simulink model "2Zad_Adasiak"  (R2020b)
settings: Solver=VariableStepAuto  StartTime=0.0  StopTime=0.0  RelTol=1e-3
undefined symbols (not defined in the file): W
libraries: CPOiS_SourcesSinks x15, CPOiS_LinearTransforms x5, CPOiS_General x1
settings Model: Creator=Krystian  LastModifiedBy=Krystian

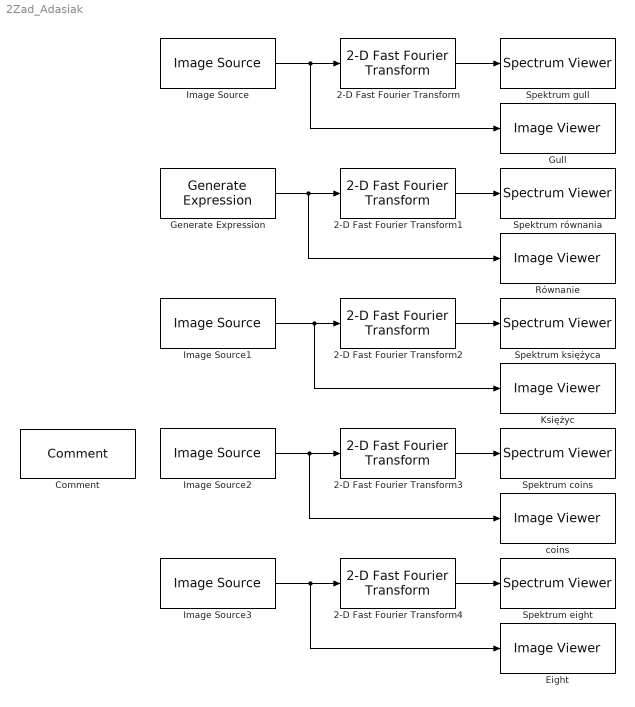
== system 2Zad_Adasiak ==
  2-D Fast Fourier Transform{,1..4} (5 alike) : CPOiS_LinearTransforms/2-D Fast Fourier Transform
      settings: SourceProductName=CPOiS - Digital image and signal processing
  Comment : CPOiS_General/Comment
      settings: SourceProductName=CPOiS - Digital image and signal processing
  Eight : CPOiS_SourcesSinks/Image Viewer
      settings: SourceProductName=CPOiS - Digital image and signal processing
  Generate Expression : CPOiS_SourcesSinks/Generate Expression  Width=256  Height=256  Expression=128.*(sin(W)+1)
      settings: SourceProductName=CPOiS - Digital image and signal processing
  Gull : CPOiS_SourcesSinks/Image Viewer
      settings: SourceProductName=CPOiS - Digital image and signal processing
  Image Source : CPOiS_SourcesSinks/Image Source  FileSelection=gull.png
      settings: SourceProductName=CPOiS - Digital image and signal processing
  Image Source1 : CPOiS_SourcesSinks/Image Source  FileSelection=moon.png
      settings: SourceProductName=CPOiS - Digital image and signal processing
  Image Source2 : CPOiS_SourcesSinks/Image Source  FileSelection=marine.png
      settings: SourceProductName=CPOiS - Digital image and signal processing
  Image Source3 : CPOiS_SourcesSinks/Image Source  FileSelection=eight.tif
      settings: SourceProductName=CPOiS - Digital image and signal processing
  Księżyc : CPOiS_SourcesSinks/Image Viewer
      settings: SourceProductName=CPOiS - Digital image and signal processing
  Równanie : CPOiS_SourcesSinks/Image Viewer
      settings: SourceProductName=CPOiS - Digital image and signal processing
  Spektrum coins : CPOiS_SourcesSinks/Spectrum Viewer
      settings: SourceProductName=CPOiS - Digital image and signal processing
  Spektrum eight : CPOiS_SourcesSinks/Spectrum Viewer
      settings: SourceProductName=CPOiS - Digital image and signal processing
  Spektrum gull : CPOiS_SourcesSinks/Spectrum Viewer
      settings: SourceProductName=CPOiS - Digital image and signal processing
  Spektrum księżyca : CPOiS_SourcesSinks/Spectrum Viewer
      settings: SourceProductName=CPOiS - Digital image and signal processing
  Spektrum równania : CPOiS_SourcesSinks/Spectrum Viewer
      settings: SourceProductName=CPOiS - Digital image and signal processing
  coins : CPOiS_SourcesSinks/Image Viewer
      settings: SourceProductName=CPOiS - Digital image and signal processing
  wires:
  2-D Fast Fourier Transform4/1 -> Spektrum eight/1
  Image Source3/1 -> Eight/1, 2-D Fast Fourier Transform4/1
  Image Source2/1 -> coins/1, 2-D Fast Fourier Transform3/1
  2-D Fast Fourier Transform1/1 -> Spektrum równania/1
  2-D Fast Fourier Transform/1 -> Spektrum gull/1
  Generate Expression/1 -> 2-D Fast Fourier Transform1/1, Równanie/1
  Image Source1/1 -> 2-D Fast Fourier Transform2/1, Księżyc/1
  2-D Fast Fourier Transform2/1 -> Spektrum księżyca/1
  Image Source/1 -> 2-D Fast Fourier Transform/1, Gull/1
  2-D Fast Fourier Transform3/1 -> Spektrum coins/1
